simulink model "main_ddp_N5"  (R2026a)
settings: Solver=VariableStepAuto  StopTime=simulation_time  FixedStep=params.MPC.dt  RelTol=1e-2
undefined symbols (not defined in the file or in its folder): params, Ref
(part 2 of 2)

== matlab function main_ddp_N5/IP_ILQR_controller_test/IP-ILQR ==
  data: x input size=params.nx; u_bar input size=[params.nu,params.MPC.N]; u1 output size=params.nu; Pd input; K0 output size=[params.nu,params.nx]; u_bar output size=[params.nu,params.MPC.N]; params parameter; x_bar_next output size=params.nx; Ref parameter; Smax input; Pb_bar output size=1; s_bar input; s_opt output; nominal_IP_Bus output Bus: nominal_IP_Bus
 function [u1,K0,u_bar, x_bar_next, Pb_bar, s_opt, nominal_IP_Bus] = ILQR(x,u_bar,Pd,params,Ref,Smax,s_bar)

% which discretization method
% D:difference, V:variational
D_method = 'D or V';
if params.D_method == 1
    D_method = 'D';       % 1:difference, 0:
    disp(D_method)
elseif params.D_method == 0
    D_method = 'V';
     % disp(D_method)
end

% 前の時間ステップからの時刻のずれを補正
u_bar(:,1:end-1) = u_bar(:,2:end);
u_bar(:,end)     = u_bar(:,end-1);
du = zeros(size(u_bar));

s_bar(:,1:end-1)   = s_bar(:,2:end);
s_bar(:,end)       = s_bar(:,end-1);

%%%%%%%%%%%%%%%%%%%%%% MPC setting %%%%%%%%%%%%%%%%%%%%%%%%%%%%%%%%%%%%%%%%
% linesearch off:0 on:1
linesearch = params.lineserch;
tsp = params.MPC.dt;            % sampling period
N = 10;                         % number of horizon 
N_iter = params.N_iter_IP;         % number of N_iter_IP

nx = size(x,1);                 
nu = size(u_bar,1);

K0 = zeros(nu,nx);             
x_bar = zeros(nx,N+1);
x_opt = zeros(nx,N+1);
du_IP = zeros(nu,N);
K0_IP = zeros(nu,nx);
x_opt_IP = zeros(nx,N+1);
du_opt = zeros(nu,N);
Qu = zeros(size(u_bar));
Qu_hat = zeros(size(u_bar));


%%%%%%%%%%%%%%%%% Interior Point setting %%%%%%%%%%%%%%%%%%%%%%%%%%%%%%%%%
mu = params.MPC.mu;
mu_iter = params.mu_iter;
mu_decrease_rate = params.mu_decrease_rate;

disp('==========================0.05s')



s_opt = zeros(size(s_bar));
c    = zeros(size(s_bar));


% 各μにおけるc,r,sの値を保存する変数
c_mu = zeros(size(c,1),size(c,2),mu_iter);  
r_mu = zeros(size(c_mu,1),size(c_mu,2),mu_iter);
s_mu = zeros(size(r_mu));
Qu_mu = zeros(size(u_bar,1),size(u_bar,2),mu_iter);
Qu_hat_mu = zeros(size(u_bar,1),size(u_bar,2),mu_iter);
%%%%%%%%%%%%%%%%% Iteration %%%%%%%%%%%%%%%%%%%%%%%%%%%%%%%%%%%%%%%%%%%%%%%
ls_gamma = 1;

for j = 1:mu_iter
   for i = 1:N_iter
        % disp('--------------') 
        if any(x_bar(1,:) < 0)
           disp(u_bar+du)
           disp(x_bar)
        end
   
        [x_bar,A,B]    = forwardpass_runge(x, u_bar, du, tsp, N, D_method,params,Ref);
        [du_opt, x_opt,s_opt,K0,ls_gamma,r] = backwardpass_IP_Quu_reg(x_bar, u_bar, du, s_bar,A,B,N,tsp,ls_gamma,Pd,params,mu,Ref,Smax);
        
        del_du = du_opt -du;
        du = du_opt;
        
        % =================================================================
        %　muの更新　
        % |F(w,s)| < 0.2*mu でN_iter の終了

        [r,Qu,Qu_hat] = F_wmu(x_opt,u_bar,du_opt,s_opt,A,B,N,Pd,params,mu,Ref,Smax);
        

        r_max = max(max(abs(r)));
        Qu_max = max(max(abs(Qu)));
        F_max = max(r_max,Qu_max);


        if r_max < mu(1)/5 && Qu_max < 1
            disp('r_max < mu/5')
            disp([j,i])
            disp([r_max,mu(1)/5])
            disp(r)
            disp(Qu)
            % Quの値があまりにも大きい場合はbreakしないようにしたい
            break
        % else
            % disp('r_max > mu/5')
            % disp([j,i])
            % disp([r_max,mu(1)/5])
            % disp(r)
        end

        % if F_max < mu(1)/5
        %     disp('F(w,mu) < mu/5')
        %     disp([j,i])
        %     disp([F_max,mu(1)/5])
        %     break
        % else
        %     disp([j,i])
        %     %disp([Qu_max,r_max])
        %     disp(del_du)
        %     disp(max(max(abs(Qu))))
        % 
        %     % if r_max > mu(1)/5
        %     %     disp('r_max > mu(1)/5')
        %     %     disp([r_max,mu(1)/5])
        %     % end
        %     % if Qu_max > mu(1)/5
        %     %     disp('Qu_max > mu(1)/5')
        %     %     disp([Qu_max,mu(1)/5])
        %     % end
        % end
        % =================================================================
   end

   
    %　各muでの r=s*c+muの計算
    for ii = 1:N
        if (x_opt(1,ii)/0.1173+params.psat/Ref.pres) < 2    
             c(:,ii) = constraints_case1(x_opt(:,ii),u_bar(:,ii),du_opt(:,ii),Pd(ii),Smax);
        else
             c(:,ii) = constraints_case2(x_opt(:,ii),u_bar(:,ii),du_opt(:,ii),Pd(ii),Smax);
        end
    end

    for ii = 1:N
        r_mu(:,ii,j)   = s_opt(:,ii).*c(:,ii)+mu;
        %r_mu(:,ii,j)   = s_opt(:,ii).*c(:,ii);
    end
    
    %  === mu毎における値の保存 ===
    c_mu(:,:,j) = c;
    s_mu(:,:,j) = s_opt;
    Qu_mu(:,:,j) = Qu;
    Qu_hat_mu(:,:,j) = Qu_hat;
    % ============================
    
    % disp(j)
    % disp(mu')
    % disp(c)
    % disp(s_opt)
    % disp(r_mu(:,:,j))
    
    % mu = mu./mu_decrease_rate;
    mu = mu/5;
    %mu(14:15) = mu(14:15)/25; 
end
% % % % % % % % % % % % % % % % % % % % % % % % % % % % % % % % % % % % % % 

Pb_bar = Pb_fun(x_bar(:,1),u_bar(:,1),du(:,1));
u1    = u_bar(:,1) + du(:,1); 
u_bar = u_bar + du;
x_bar_next = x_opt(:,2);




nominal_IP_Bus.u_b = u_bar;
nominal_IP_Bus.du = du;
nominal_IP_Bus.K0 = K0;
nominal_IP_Bus.x_opt = x_opt;
nominal_IP_Bus.s = s_opt;
nominal_IP_Bus.c = c;
nominal_IP_Bus.Qu = Qu;
nominal_IP_Bus.Qu_hat = Qu_hat;
nominal_IP_Bus.r = r_mu(:,:,end); % r_muはmuごとのrの値が入っている．その最後の値（イテレーションの最後）を保存
end
